simulink model "Single_Axis_Pitch_Disturbance"  (R2024b)
settings: Solver=ode4  StartTime=0.0  StopTime=0.2  FixedStep=0.001  RelTol=1e-3
settings Model: Creator=Zohaib  LastModifiedBy=Zohaib
settings DataIOCC: ReturnWorkspaceOutputs=off

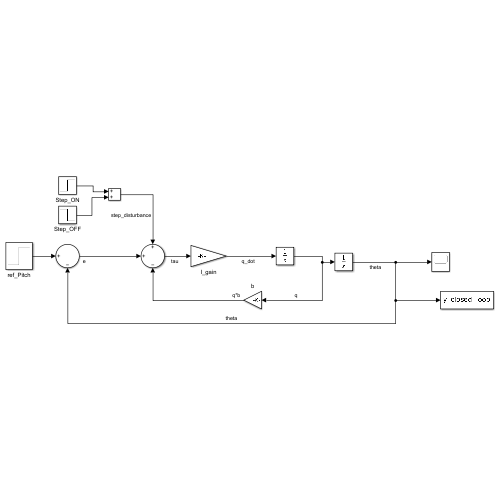
[thumbnail: Simulink's stored preview of the top-level diagram]
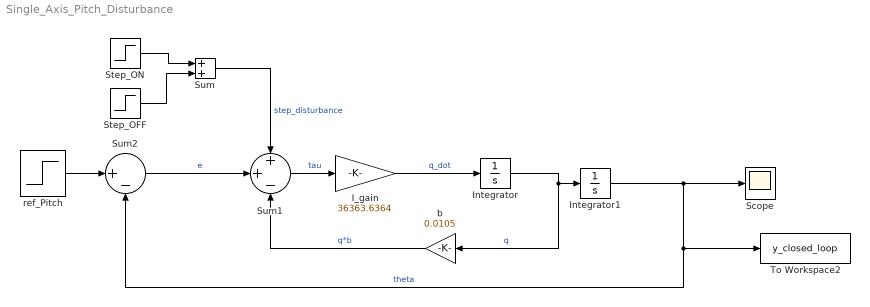
== system Single_Axis_Pitch_Disturbance ==
  I_gain : Gain  Gain=36363.6364
  Integrator : Integrator
  Integrator1 : Integrator
  Scope : Scope
  Step_OFF : Step  Time=0.0735  After=-0.0003  SampleTime=0.001
  Step_ON : Step  Time=0.07  After=0.0003  SampleTime=0.001
  Sum : Sum
  Sum1 : Sum  Inputs=++-
  Sum2 : Sum  Inputs=|+-
  To Workspace2 : ToWorkspace  VariableName=y_closed_loop  SaveFormat=Timeseries  SampleTime=-1
  b : Gain  Gain=0.0105
  ref_Pitch : Step  Time=0  After=5*(pi/180)  SampleTime=0.001
  wires:
  Integrator1/1 -> Scope/1, To Workspace2/1, Sum2/2  "theta"
  Integrator/1 -> b/1, Integrator1/1  "q"
  I_gain/1 -> Integrator/1  "q_dot"
  ref_Pitch/1 -> Sum2/1
  Sum1/1 -> I_gain/1  "tau"
  Step_ON/1 -> Sum/1
  Step_OFF/1 -> Sum/2
  Sum/1 -> Sum1/1  "step_disturbance"
  Sum2/1 -> Sum1/2  "e"
  b/1 -> Sum1/3  "q*b"
